simulink model "P3"  (R2019a)
settings: Solver=VariableStepAuto  StartTime=0.0  StopTime=50.0  RelTol=1e-3
settings Model: Creator=ADMIN  LastModifiedBy=ADMIN

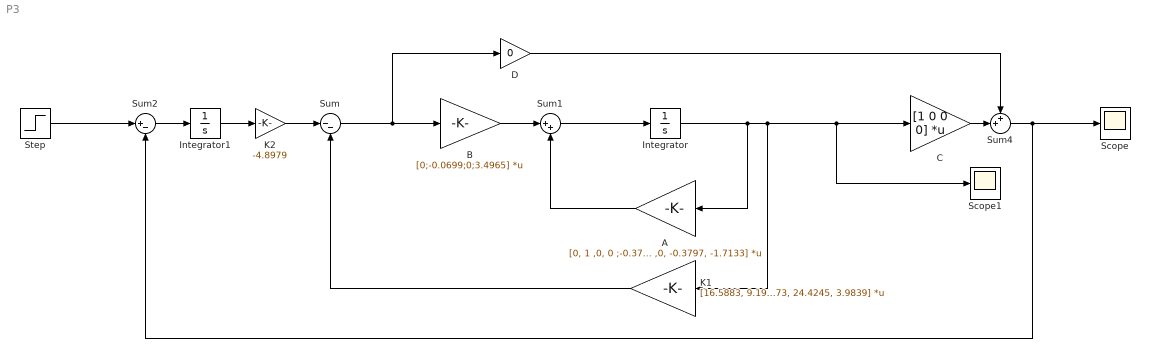
== system P3 ==
  A : Gain  Gain=[0, 1 ,0, 0 ;-0.378 ,0 ,7.0147 ,0.0343;0, 0, 0, 1; 18.9001 ,0, -0.3797, -1.7133]  Multiplication=Matrix(K*u) (u vector)
  B : Gain  Gain=[0;-0.0699;0;3.4965]  Multiplication=Matrix(K*u) (u vector)
  C : Gain  Gain=[1 0 0 0]  Multiplication=Matrix(K*u) (u vector)
  D : Gain  Gain=0
  Integrator : Integrator
  Integrator1 : Integrator
  K1 : Gain  Gain=[16.5883, 9.1973, 24.4245, 3.9839]  Multiplication=Matrix(K*u) (u vector)
  K2 : Gain  Gain=-4.8979
  Scope : Scope
  Scope1 : Scope
  Step : Step  Time=0  After=0.1  SampleTime=0
  Sum : Sum  Inputs=|--
  Sum1 : Sum  Inputs=|++
  Sum2 : Sum  Inputs=|+-
  Sum4 : Sum  Inputs=++|
  wires:
  Sum4/1 -> Sum2/2, Scope/1
  K1/1 -> Sum/2
  C/1 -> Sum4/2
  D/1 -> Sum4/1
  A/1 -> Sum1/2
  Sum/1 -> B/1, D/1
  B/1 -> Sum1/1
  Sum1/1 -> Integrator/1
  K2/1 -> Sum/1
  Integrator1/1 -> K2/1
  Sum2/1 -> Integrator1/1
  Step/1 -> Sum2/1
  Integrator/1 -> C/1, Scope1/1, K1/1, A/1
